simulink model "IF"  (R2024a)
settings: Solver=FixedStepAuto  StartTime=0.0  StopTime=5  FixedStep=1e-4  RelTol=1e-3
values from neighbouring files (symbols this model uses):
  Kt = 0.132    [IF.sldd]
  Pn = 8.0    [IF.sldd]
  Udc = 48.0    [IF.sldd]
undefined symbols (not defined in the file or in its folder): curr_d_ki, curr_d_kp, curr_q_ki, curr_q_kp, DiscIntNeverNeededParam
libraries: slpidlib x6, mcbplantlib x3, autolibpmsmexterior x3
(part 1 of 2)
settings Model: DataDictionary=IF.sldd  Creator=Administrator  LastModifiedBy=WuHongrui
settings OptimizationCC: DefaultParameterBehavior=Inlined  UseDivisionForNetSlopeComputation=on  GainParamInheritBuiltInType=on  UseFloatMulNetSlope=on  InlineInvariantSignals=on  PassReuseOutputArgsAs=Individual arguments  ZeroExternalMemoryAtStartup=off  ZeroInternalMemoryAtStartup=off  NoFixptDivByZeroProtection=on  EfficientFloat2IntCast=on  LifeSpan=1  OptimizeBlockOrder=speed  DifferentSizesBufferReuse=on  EfficientTunableParamExpr=on
settings DebuggingCC: ParameterTunabilityLossMsg=error  UnconnectedInputMsg=warning  UnconnectedOutputMsg=warning  UnconnectedLineMsg=warning
settings HardwareCC: ProdBitPerPointer=32  ProdBitPerSizeT=32  ProdBitPerPtrDiffT=32  ProdLargestAtomicInteger=Long  ProdLargestAtomicFloat=Double  ProdWordSize=32  ProdLongLongMode=on  ProdHWDeviceType=ARM Compatible->ARM Cortex-M
settings ModelReferenceCC: EnableRefExpFcnMdlSchedulingChecks=on
settings SFSimCC: MATLABDynamicMemAlloc=off
settings RTWCC: Description=Embedded Coder  SystemTargetFile=ert.tlc  GenCodeOnly=on  TemplateMakefile=ert_default_tmf  GenerateReport=on  LaunchReport=on  GenerateCodeReplacementReport=on  GPUComputeCapability=3.5  DLArmComputeVersion=19.05
settings CodeAppCC: ForceParamTrailComments=on  IgnoreCustomStorageClasses=off  OperatorAnnotations=on  SimulinkDataObjDesc=on  SFDataObjDesc=on  CustomSymbolStrGlobalVar=rt$N$M  CustomSymbolStrType=$N$M  CustomSymbolStrFcn=$N$M$F  CustomSymbolStrMacro=$N$M  InsertBlockDesc=on
settings ERTTargetCC: TargetLangStandard=C99 (ISO)  CodeReplacementLibrary=ARM Cortex-M  IncludeMdlTerminateFcn=off  CombineSignalStateStructs=on  SupportComplex=off  SupportNonInlinedSFcns=on  InlinedParameterPlacement=NonHierarchical  ERTCustomFileTemplate=example_file_process.tlc  ERTFilePackagingFormat=CompactWithDataFile

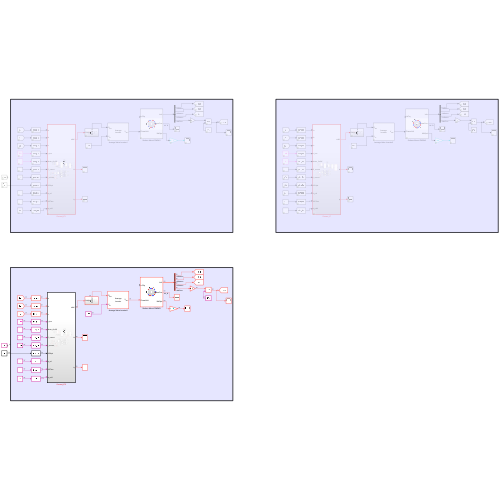
[thumbnail: Simulink's stored preview of the top-level diagram]
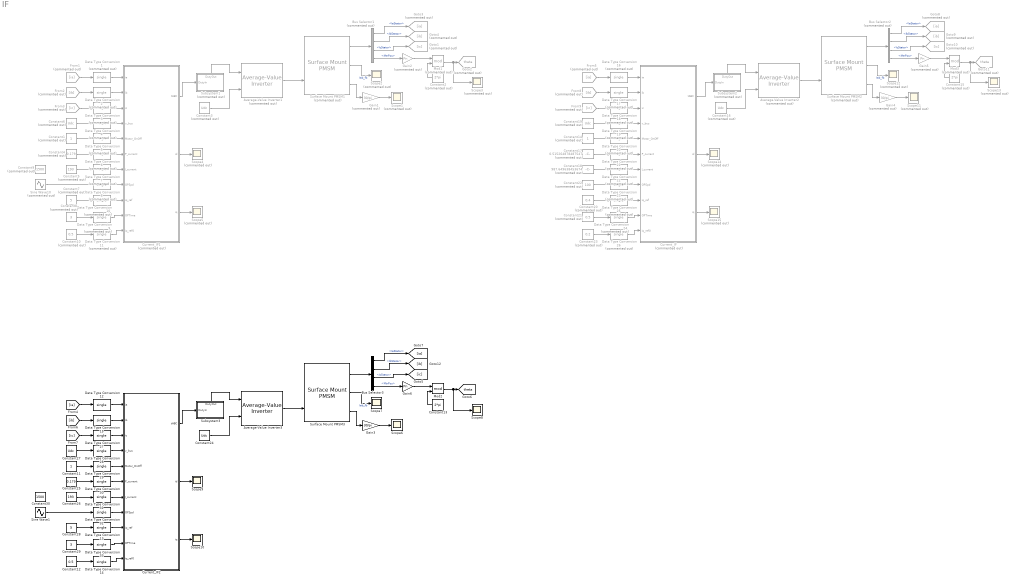
== system IF ==
  Average-Value Inverter1 : mcbplantlib/Average-Value Inverter  Commented=on
  Average-Value Inverter2 : mcbplantlib/Average-Value Inverter  Commented=on
  Average-Value Inverter3 : mcbplantlib/Average-Value Inverter
  Bus Selector1 : BusSelector  Commented=on  OutputSignals=IaStator,IbStator,IcStator,MtrPos
  Bus Selector2 : BusSelector  Commented=on  OutputSignals=IaStator,IbStator,IcStator,MtrPos
  Bus Selector3 : BusSelector  OutputSignals=IaStator,IbStator,IcStator,MtrPos
  Constant1 : Constant  Commented=on  OutDataTypeStr=single
  Constant10 : Constant  Commented=on  Value=0.5  OutDataTypeStr=single
  Constant11 : Constant  OutDataTypeStr=single
  Constant12 : Constant  Value=0.5  OutDataTypeStr=single
  Constant13 : Constant  Value=2*pi  OutDataTypeStr=single
  Constant14 : Constant  Commented=on  OutDataTypeStr=single
  Constant15 : Constant  Commented=on  Value=2*pi  OutDataTypeStr=single
  Constant16 : Constant  Commented=on  Value=Udc
  Constant17 : Constant  Commented=on  Value=0.515264878487547  OutDataTypeStr=single
  Constant18 : Constant  Commented=on  Value=987.649638453674  OutDataTypeStr=single
  Constant19 : Constant  Commented=on  Value=Udc  OutDataTypeStr=single
  Constant2 : Constant  Commented=on  Value=2*pi  OutDataTypeStr=single
  Constant20 : Constant  Commented=on  Value=0.4  OutDataTypeStr=single
  Constant21 : Constant  Commented=on  Value=0.5  OutDataTypeStr=single
  Constant22 : Constant  Commented=on  Value=100  OutDataTypeStr=single
  Constant23 : Constant  Commented=on  Value=0.2  OutDataTypeStr=single
  Constant24 : Constant  Value=Udc
  Constant25 : Constant  Value=0.179  OutDataTypeStr=single
  Constant26 : Constant  Value=193  OutDataTypeStr=single
  Constant27 : Constant  Value=Udc  OutDataTypeStr=single
  Constant28 : Constant  Value=5  OutDataTypeStr=single
  Constant29 : Constant  Value=3  OutDataTypeStr=single
  Constant3 : Constant  Commented=on  Value=Udc
  Constant30 : Constant  Value=1500  OutDataTypeStr=single
  Constant4 : Constant  Commented=on  Value=0.179  OutDataTypeStr=single
  Constant5 : Constant  Commented=on  Value=193  OutDataTypeStr=single
  Constant6 : Constant  Commented=on  Value=Udc  OutDataTypeStr=single
  Constant7 : Constant  Commented=on  Value=5  OutDataTypeStr=single
  Constant8 : Constant  Commented=on  Value=3  OutDataTypeStr=single
  Constant9 : Constant  Commented=on  Value=1500  OutDataTypeStr=single
  Current_IF : Subsystem  Commented=on  TreatAsAtomicUnit=on
  Current_IF1 : Subsystem  Commented=on  TreatAsAtomicUnit=on
  Current_IF2 : Subsystem  TreatAsAtomicUnit=on
  Data Type Conversion{1..11,16..26} (22 alike) : DataTypeConversion  Commented=on  OutDataTypeStr=single  SaturateOnIntegerOverflow=off  RndMeth=Floor
  Data Type Conversion{12..15,27..33} (11 alike) : DataTypeConversion  OutDataTypeStr=single  SaturateOnIntegerOverflow=off  RndMeth=Floor
  From1 : From  Commented=on  GotoTag=ia
  From2 : From  Commented=on  GotoTag=ib
  From3 : From  Commented=on  GotoTag=ic
  From5 : From  Commented=on  GotoTag=ia
  From8 : From  Commented=on  GotoTag=ib
  From9 : From  Commented=on  GotoTag=ic
  Gain1 : Gain  Commented=on  Gain=30/pi  OutDataTypeStr=single
  Gain2 : Gain  Commented=on  Gain=Pn  OutDataTypeStr=single
  Gain3 : Gain  Gain=30/pi  OutDataTypeStr=single
  Gain4 : Gain  Commented=on  Gain=30/pi  OutDataTypeStr=single
  Gain5 : Gain  Commented=on  Gain=Pn  OutDataTypeStr=single
  Gain6 : Gain  Gain=Pn  OutDataTypeStr=single
  Goto1 : Goto  Commented=on  GotoTag=ic
  Goto10 : Goto  Commented=on  GotoTag=ic
  Goto11 : Goto  Commented=on  GotoTag=theta  TagVisibility=global
  Goto2 : Goto  Commented=on  GotoTag=theta  TagVisibility=global
  Goto3 : Goto  Commented=on  GotoTag=ia
  Goto4 : Goto  Commented=on  GotoTag=ib
  Goto8 : Goto  Commented=on  GotoTag=ia
  Goto9 : Goto  Commented=on  GotoTag=ib
  Mod1 : Math  Commented=on  Operator=mod  OutputSignalType=real
  Mod2 : Math  Operator=mod  OutputSignalType=real
  Mod3 : Math  Commented=on  Operator=mod  OutputSignalType=real
  Scope{1..5,11..15} (10 alike) : Scope  Commented=on
  Scope{6..10} (5 alike) : Scope
  Sine Wave1 : Sin  Amplitude=500  Frequency=5  SampleTime=0
  Sine Wave10 : Sin  Commented=on  Amplitude=500  Frequency=5  SampleTime=0
  Subsystem1 : Subsystem  Commented=on
      settings: PortSchema="{\"entries\":[{\"content\":{\"sides\":[{\"content\":{\"connectorIds\":[\"In1\"]},\"type\":\"ConnectorPlacement.EquallySpacedRectSide\",\"uuid\":\"8ccc51de-fa2a-4900-80a3-4cdf9aa76f01\"},{\"content\":{\"connectorIds\":[],\"side\":\"RIGHT\"},\"type\":\"ConnectorPlacement.EquallySpacedRectSide\",\"uuid\":\"32c06e0d-3f1d-4948-af96-e310e54308a0\"},{\"content\":{\"connectorIds\":[\"Out1\"],\"side\":\"TOP\"},\"type\":\"ConnectorPlacement.EquallySpacedRectSide\",\"uuid\":\"a9066067-2c54-42a8-b4d7-fb86ac71b860\"}]},\"type\":\"ConnectorPlacement.EquallySpacedConnector\",\"uuid\":\"e4576975-acad-4e16-822f-2c2e7f23d7a7\"}],\"packageUris\":[\"http://schema.mathworks.com/mf0/Connector/R2020b\"],\"version\":\"1.0\"}"
  Subsystem2 : Subsystem  Commented=on
      settings: PortSchema="{\"entries\":[{\"content\":{\"sides\":[{\"content\":{\"connectorIds\":[\"In1\"]},\"type\":\"ConnectorPlacement.EquallySpacedRectSide\",\"uuid\":\"8ccc51de-fa2a-4900-80a3-4cdf9aa76f01\"},{\"content\":{\"connectorIds\":[],\"side\":\"RIGHT\"},\"type\":\"ConnectorPlacement.EquallySpacedRectSide\",\"uuid\":\"32c06e0d-3f1d-4948-af96-e310e54308a0\"},{\"content\":{\"connectorIds\":[\"Out1\"],\"side\":\"TOP\"},\"type\":\"ConnectorPlacement.EquallySpacedRectSide\",\"uuid\":\"a9066067-2c54-42a8-b4d7-fb86ac71b860\"}]},\"type\":\"ConnectorPlacement.EquallySpacedConnector\",\"uuid\":\"e4576975-acad-4e16-822f-2c2e7f23d7a7\"}],\"packageUris\":[\"http://schema.mathworks.com/mf0/Connector/R2020b\"],\"version\":\"1.0\"}"
  Subsystem3 : Subsystem
      settings: PortSchema="{\"entries\":[{\"content\":{\"sides\":[{\"content\":{\"connectorIds\":[\"In1\"]},\"type\":\"ConnectorPlacement.EquallySpacedRectSide\",\"uuid\":\"8ccc51de-fa2a-4900-80a3-4cdf9aa76f01\"},{\"content\":{\"connectorIds\":[],\"side\":\"RIGHT\"},\"type\":\"ConnectorPlacement.EquallySpacedRectSide\",\"uuid\":\"32c06e0d-3f1d-4948-af96-e310e54308a0\"},{\"content\":{\"connectorIds\":[\"Out1\"],\"side\":\"TOP\"},\"type\":\"ConnectorPlacement.EquallySpacedRectSide\",\"uuid\":\"a9066067-2c54-42a8-b4d7-fb86ac71b860\"}]},\"type\":\"ConnectorPlacement.EquallySpacedConnector\",\"uuid\":\"e4576975-acad-4e16-822f-2c2e7f23d7a7\"}],\"packageUris\":[\"http://schema.mathworks.com/mf0/Connector/R2020b\"],\"version\":\"1.0\"}"
  Surface Mount PMSM1 : autolibpmsmexterior/Surface Mount PMSM  Commented=on  port_config=Torque  sim_type=Discrete  Ts=1e-4  P=Pn  Rs=Rs  Ldq_=L  KConstText=Torque constant (Kt):  lambda_pm=flux  Ke=0.0059268  Kt=Kt  mechanical=[0.096e-4, 2e-5, 0]  idq0=[0 0]  theta_init=0  omega_init=0  KConst=Kt  lambda_pm_calc=0.011  RefBlkName='autolibpmsmexterior/Surface Mount PMSM'  aMode=5  Ldq="[0.0017      0.0017]"
  Surface Mount PMSM2 : autolibpmsmexterior/Surface Mount PMSM  Commented=on  port_config=Torque  sim_type=Discrete  Ts=1e-4  P=Pn  Rs=Rs  Ldq_=L  KConstText=Torque constant (Kt):  lambda_pm=flux  Ke=0.0059268  Kt=Kt  mechanical=[0.096e-4, 2e-5, 0]  idq0=[0 0]  theta_init=0  omega_init=0  KConst=Kt  lambda_pm_calc=0.011  RefBlkName='autolibpmsmexterior/Surface Mount PMSM'  aMode=5  Ldq="[0.0017      0.0017]"
  Surface Mount PMSM3 : autolibpmsmexterior/Surface Mount PMSM  port_config=Torque  sim_type=Discrete  Ts=1e-4  P=Pn  Rs=Rs  Ldq_=L  KConstText=Torque constant (Kt):  lambda_pm=flux  Ke=0.0059268  Kt=Kt  mechanical=[0.096e-4, 2e-5, 0]  idq0=[0 0]  theta_init=0  omega_init=0  KConst=Kt  lambda_pm_calc=0.011  RefBlkName='autolibpmsmexterior/Surface Mount PMSM'  aMode=5  Ldq="[0.0017      0.0017]"
  tag scope: theta=global
  wires:
  Data Type Conversion18/1 -> Current_IF/3(ic)
  Current_IF/3(iq) -> Scope15/1
  Gain4/1 -> Scope11/1
  Constant16/1 -> Average-Value Inverter2/2
  From8/1 -> Data Type Conversion17/1
  Data Type Conversion16/1 -> Current_IF/1(ia)
  Bus Selector2/4 -> Gain5/1  "<MtrPos>"
  Constant17/1 -> Data Type Conversion21/1
  Constant18/1 -> Data Type Conversion22/1
  Data Type Conversion19/1 -> Current_IF/4(v_bus)
  Constant19/1 -> Data Type Conversion19/1
  Data Type Conversion21/1 -> Current_IF/6(P_current)
  Current_IF/2(id) -> Scope14/1
  Current_IF/1(tABC) -> Subsystem2/1(DutyIn)
  Data Type Conversion20/1 -> Current_IF/5(Motor_OnOff)
  Data Type Conversion22/1 -> Current_IF/7(I_current)
  Bus Selector2/1 -> Goto8/1  "<IaStator>"
  Average-Value Inverter2/1 -> Surface Mount PMSM2/2
  From9/1 -> Data Type Conversion18/1
  Bus Selector2/2 -> Goto9/1  "<IbStator>"
  Constant14/1 -> Data Type Conversion20/1
  Subsystem2/1(DutyOut) -> Average-Value Inverter2/1
  Constant15/1 -> Mod3/2
  Mod3/1 -> Scope13/1, Goto11/1
  From5/1 -> Data Type Conversion16/1
  Surface Mount PMSM2/3 -> Gain4/1
  Gain5/1 -> Mod3/1
  Bus Selector2/3 -> Goto10/1  "<IcStator>"
  Surface Mount PMSM2/1 -> Bus Selector2/1
  Data Type Conversion17/1 -> Current_IF/2(ib)
  Surface Mount PMSM2/2 -> Scope12/1  "Iab_fb"
  Data Type Conversion23/1 -> Current_IF/8(OPSpd)
  Constant22/1 -> Data Type Conversion23/1
  Data Type Conversion25/1 -> Current_IF/9(iq_ref)
  Constant20/1 -> Data Type Conversion25/1
  Constant21/1 -> Data Type Conversion24/1
  Data Type Conversion24/1 -> Current_IF/10(OPTime)
  Constant23/1 -> Data Type Conversion26/1
  Data Type Conversion26/1 -> Current_IF/11(iq_ref0)
  Current_IF1/1(tABC) -> Subsystem1/1(DutyIn)
  Bus Selector1/2 -> Goto4/1  "<IbStator>"
  Gain1/1 -> Scope1/1
  Data Type Conversion3/1 -> Current_IF1/3(ic)
  From2/1 -> Data Type Conversion2/1
  Constant3/1 -> Average-Value Inverter1/2
  Constant1/1 -> Data Type Conversion5/1
  Constant5/1 -> Data Type Conversion7/1
  Current_IF1/2(id) -> Scope4/1
  Constant4/1 -> Data Type Conversion6/1
  Data Type Conversion6/1 -> Current_IF1/6(P_current)
  Bus Selector1/4 -> Gain2/1  "<MtrPos>"
  Data Type Conversion1/1 -> Current_IF1/1(ia)
  Current_IF1/3(iq) -> Scope5/1
  From3/1 -> Data Type Conversion3/1
  Surface Mount PMSM1/3 -> Gain1/1
  Constant10/1 -> Data Type Conversion11/1
  Bus Selector1/1 -> Goto3/1  "<IaStator>"
  Average-Value Inverter1/1 -> Surface Mount PMSM1/2
  Constant2/1 -> Mod1/2
  Constant7/1 -> Data Type Conversion10/1
  Data Type Conversion5/1 -> Current_IF1/5(Motor_OnOff)
  Constant8/1 -> Data Type Conversion9/1
  Data Type Conversion8/1 -> Current_IF1/8(OPSpd)
  Gain2/1 -> Mod1/1
  Data Type Conversion2/1 -> Current_IF1/2(ib)
  Surface Mount PMSM1/2 -> Scope2/1  "Iab_fb"
  Subsystem1/1(DutyOut) -> Average-Value Inverter1/1
  Data Type Conversion10/1 -> Current_IF1/9(iq_ref)
  Data Type Conversion7/1 -> Current_IF1/7(I_current)
  Data Type Conversion4/1 -> Current_IF1/4(v_bus)
  Constant6/1 -> Data Type Conversion4/1
  Sine Wave10/1 -> Data Type Conversion8/1
  Bus Selector1/3 -> Goto1/1  "<IcStator>"
  Data Type Conversion9/1 -> Current_IF1/10(OPTime)
  Surface Mount PMSM1/1 -> Bus Selector1/1
  Mod1/1 -> Scope3/1, Goto2/1
  Data Type Conversion11/1 -> Current_IF1/11(iq_ref0)
  From1/1 -> Data Type Conversion1/1
  Constant11/1 -> Data Type Conversion29/1
  Constant26/1 -> Data Type Conversion31/1
  Constant25/1 -> Data Type Conversion30/1
  Data Type Conversion27/1 -> Current_IF2/3(ic)
  Surface Mount PMSM3/1 -> Bus Selector3/1
  [ib] -> Data Type Conversion15/1
  Data Type Conversion14/1 -> Current_IF2/11(iq_ref0)
  Data Type Conversion12/1 -> Current_IF2/1(ia)
  Mod2/1 -> Scope8/1, [theta]
  Subsystem3/1(DutyOut) -> Average-Value Inverter3/1
  Constant28/1 -> Data Type Conversion13/1
  Data Type Conversion33/1 -> Current_IF2/10(OPTime)
  Constant13/1 -> Mod2/2
  [ia] -> Data Type Conversion12/1
  Bus Selector3/3 -> [ic]  "<IcStator>"
  Current_IF2/2(id) -> Scope9/1
  Current_IF2/3(iq) -> Scope10/1
  Sine Wave1/1 -> Data Type Conversion32/1
  Current_IF2/1(tABC) -> Subsystem3/1(DutyIn)
  Constant27/1 -> Data Type Conversion28/1
  Data Type Conversion15/1 -> Current_IF2/2(ib)
  Surface Mount PMSM3/2 -> Scope7/1  "Iab_fb"
  Data Type Conversion30/1 -> Current_IF2/6(P_current)
  Constant24/1 -> Average-Value Inverter3/2
  Bus Selector3/4 -> Gain6/1  "<MtrPos>"
  Bus Selector3/2 -> [ib]  "<IbStator>"
  [ic] -> Data Type Conversion27/1
  Gain6/1 -> Mod2/1
  Data Type Conversion28/1 -> Current_IF2/4(v_bus)
  Constant29/1 -> Data Type Conversion33/1
  Constant12/1 -> Data Type Conversion14/1
  Data Type Conversion29/1 -> Current_IF2/5(Motor_OnOff)
  Surface Mount PMSM3/3 -> Gain3/1
  Bus Selector3/1 -> [ia]  "<IaStator>"
  Average-Value Inverter3/1 -> Surface Mount PMSM3/2
  Gain3/1 -> Scope6/1
  Data Type Conversion32/1 -> Current_IF2/8(OPSpd)
  Data Type Conversion31/1 -> Current_IF2/7(I_current)
  Data Type Conversion13/1 -> Current_IF2/9(iq_ref)

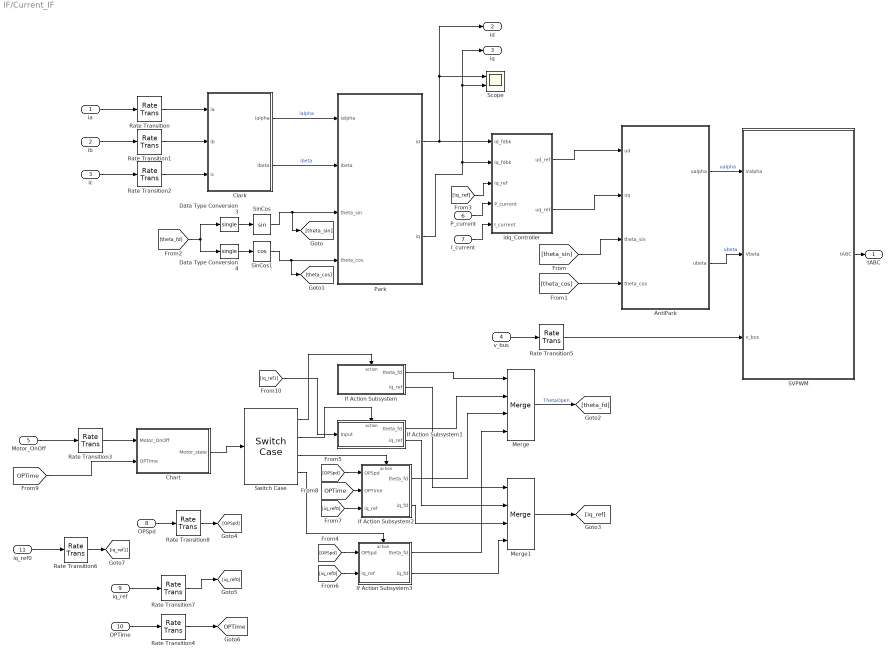
== system IF/Current_IF ==
  ia : Inport
  ib : Inport  Port=2
  ic : Inport  Port=3
  v_bus : Inport  Port=4
  Motor_OnOff : Inport  Port=5
  P_current : Inport  Port=6
  I_current : Inport  Port=7
  OPSpd : Inport  Port=8
  iq_ref : Inport  Port=9
  OPTime : Inport  Port=10
  iq_ref0 : Inport  Port=11
  AntiPark : Subsystem
  Chart : Stateflow chart  TreatAsAtomicUnit=on
  Clark : Subsystem
  Data Type Conversion3 : DataTypeConversion  OutDataTypeStr=single  SaturateOnIntegerOverflow=off  RndMeth=Floor
  Data Type Conversion4 : DataTypeConversion  OutDataTypeStr=single  SaturateOnIntegerOverflow=off  RndMeth=Floor
  If Action Subsystem : Subsystem  TreatAsAtomicUnit=on
  If Action Subsystem1 : Subsystem  TreatAsAtomicUnit=on
  If Action Subsystem2 : Subsystem  TreatAsAtomicUnit=on
  If Action Subsystem3 : Subsystem  TreatAsAtomicUnit=on
  Merge : Merge  Inputs=4
  Merge1 : Merge  Inputs=4
  Park : Subsystem
  Rate Transition{,1..8} (9 alike) : RateTransition
  SVPWM : Subsystem  TreatAsAtomicUnit=on
  Scope : Scope  NumInputPorts=2
  SinCos : Trigonometry
  SinCos1 : Trigonometry  Operator=cos
  Switch Case : SwitchCase  CaseConditions={1,2,3,4}  ShowDefaultCase=off
  idq_Controller : Subsystem
  tABC : Outport
  id : Outport  Port=2
  iq : Outport  Port=3
  tag scope: OPTime=global
  wires:
  Data Type Conversion4/1 -> SinCos1/1
  Data Type Conversion3/1 -> SinCos/1
  AntiPark/2(ubeta) -> SVPWM/2(Vbeta)  "ubeta"
  AntiPark/1(ualpha) -> SVPWM/1(Valpha)  "ualpha"
  [theta_cos] -> AntiPark/4(theta_cos)
  [theta_sin] -> AntiPark/3(theta_sin)
  SinCos/1 -> Park/3(theta_sin), [theta_sin]
  [theta_fd] -> Data Type Conversion3/1, Data Type Conversion4/1
  SinCos1/1 -> Park/4(theta_cos), [theta_cos]
  v_bus/1 -> Rate Transition5/1
  SVPWM/1(tABC) -> tABC/1
  ib/1 -> Rate Transition1/1
  ia/1 -> Rate Transition/1
  ic/1 -> Rate Transition2/1
  Clark/1(ialpha) -> Park/1(ialpha)  "ialpha"
  Clark/2(ibeta) -> Park/2(ibeta)  "ibeta"
  idq_Controller/1(ud_ref) -> AntiPark/1(ud)
  idq_Controller/2(uq_ref) -> AntiPark/2(uq)
  Park/1(id) -> id/1, Scope/1, idq_Controller/1(id_fdbk)
  Park/2(iq) -> Scope/2, iq/1, idq_Controller/2(iq_fdbk)
  [iq_ref] -> idq_Controller/3(iq_ref)
  [OPSpd] -> If Action Subsystem2/1(OPSpd)
  [iq_ref0] -> If Action Subsystem3/2(iq_ref)
  Switch Case/2 -> If Action Subsystem1/Action
  Chart/1(Motor_state) -> Switch Case/1
  [OPSpd] -> If Action Subsystem3/1(OPSpd)
  Switch Case/4 -> If Action Subsystem3/Action
  [OPTime] -> If Action Subsystem2/2(OPTime)
  [iq_ref0] -> If Action Subsystem2/3(iq_ref)
  Switch Case/1 -> If Action Subsystem/Action
  Switch Case/3 -> If Action Subsystem2/Action
  If Action Subsystem/1(theta_fd) -> Merge/1
  If Action Subsystem1/1(theta_fd) -> Merge/2
  If Action Subsystem2/1(theta_fd) -> Merge/3
  If Action Subsystem3/1(theta_fd) -> Merge/4
  If Action Subsystem/2(iq_ref) -> Merge1/1
  If Action Subsystem1/2(iq_ref) -> Merge1/2
  If Action Subsystem2/2(iq_fd) -> Merge1/3
  If Action Subsystem3/2(iq_fd) -> Merge1/4
  Merge/1 -> [theta_fd]  "ThetaOpen"
  Merge1/1 -> [iq_ref]
  Motor_OnOff/1 -> Rate Transition3/1
  P_current/1 -> idq_Controller/4(P_current)
  I_current/1 -> idq_Controller/5(I_current)
  Rate Transition/1 -> Clark/1(ia)
  Rate Transition1/1 -> Clark/2(ib)
  Rate Transition2/1 -> Clark/3(ic)
  Rate Transition5/1 -> SVPWM/3(v_bus)
  OPTime/1 -> Rate Transition4/1
  Rate Transition3/1 -> Chart/1(Motor_OnOff)
  Rate Transition4/1 -> [OPTime]
  [OPTime] -> Chart/2(OPTime)
  iq_ref0/1 -> Rate Transition6/1
  [iq_ref1] -> If Action Subsystem1/1(Input)
  Rate Transition6/1 -> [iq_ref1]
  iq_ref/1 -> Rate Transition7/1
  Rate Transition7/1 -> [iq_ref0]
  Rate Transition8/1 -> [OPSpd]
  OPSpd/1 -> Rate Transition8/1

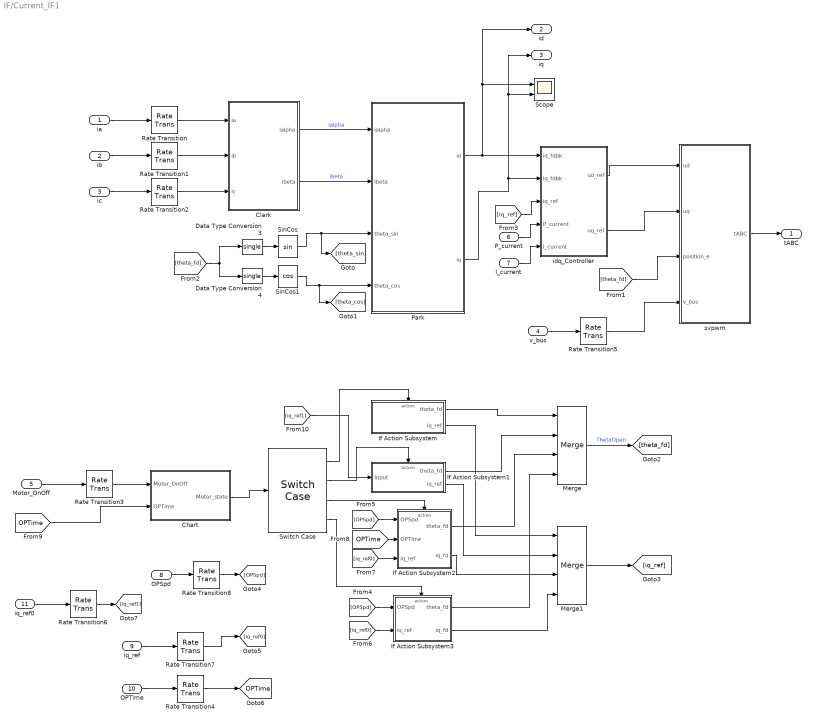
== system IF/Current_IF1 ==
  ia : Inport
  ib : Inport  Port=2
  ic : Inport  Port=3
  v_bus : Inport  Port=4
  Motor_OnOff : Inport  Port=5
  P_current : Inport  Port=6
  I_current : Inport  Port=7
  OPSpd : Inport  Port=8
  iq_ref : Inport  Port=9
  OPTime : Inport  Port=10
  iq_ref0 : Inport  Port=11
  Chart : Stateflow chart  TreatAsAtomicUnit=on
  Clark : Subsystem
  Data Type Conversion3 : DataTypeConversion  OutDataTypeStr=single  SaturateOnIntegerOverflow=off  RndMeth=Floor
  Data Type Conversion4 : DataTypeConversion  OutDataTypeStr=single  SaturateOnIntegerOverflow=off  RndMeth=Floor
  If Action Subsystem : Subsystem  TreatAsAtomicUnit=on
  If Action Subsystem1 : Subsystem  TreatAsAtomicUnit=on
  If Action Subsystem2 : Subsystem  TreatAsAtomicUnit=on
  If Action Subsystem3 : Subsystem  TreatAsAtomicUnit=on
  Merge : Merge  Inputs=4
  Merge1 : Merge  Inputs=4
  Park : Subsystem
  Rate Transition{,1..8} (9 alike) : RateTransition
  Scope : Scope  NumInputPorts=2
  SinCos : Trigonometry
  SinCos1 : Trigonometry  Operator=cos
  Switch Case : SwitchCase  CaseConditions={1,2,3,4}  ShowDefaultCase=off
  idq_Controller : Subsystem
  svpwm : Subsystem
  tABC : Outport
  id : Outport  Port=2
  iq : Outport  Port=3
  tag scope: OPTime=global
  wires:
  Data Type Conversion4/1 -> SinCos1/1
  Data Type Conversion3/1 -> SinCos/1
  SinCos/1 -> Park/3(theta_sin), [theta_sin]
  [theta_fd] -> Data Type Conversion3/1, Data Type Conversion4/1
  SinCos1/1 -> Park/4(theta_cos), [theta_cos]
  v_bus/1 -> Rate Transition5/1
  ib/1 -> Rate Transition1/1
  ia/1 -> Rate Transition/1
  ic/1 -> Rate Transition2/1
  Clark/1(ialpha) -> Park/1(ialpha)  "ialpha"
  Clark/2(ibeta) -> Park/2(ibeta)  "ibeta"
  Park/1(id) -> id/1, Scope/1, idq_Controller/1(id_fdbk)
  Park/2(iq) -> Scope/2, iq/1, idq_Controller/2(iq_fdbk)
  [iq_ref] -> idq_Controller/3(iq_ref)
  [OPSpd] -> If Action Subsystem2/1(OPSpd)
  [iq_ref0] -> If Action Subsystem3/2(iq_ref)
  Switch Case/2 -> If Action Subsystem1/Action
  Chart/1(Motor_state) -> Switch Case/1
  [OPSpd] -> If Action Subsystem3/1(OPSpd)
  Switch Case/4 -> If Action Subsystem3/Action
  [OPTime] -> If Action Subsystem2/2(OPTime)
  [iq_ref0] -> If Action Subsystem2/3(iq_ref)
  Switch Case/1 -> If Action Subsystem/Action
  Switch Case/3 -> If Action Subsystem2/Action
  If Action Subsystem/1(theta_fd) -> Merge/1
  If Action Subsystem1/1(theta_fd) -> Merge/2
  If Action Subsystem2/1(theta_fd) -> Merge/3
  If Action Subsystem3/1(theta_fd) -> Merge/4
  If Action Subsystem/2(iq_ref) -> Merge1/1
  If Action Subsystem1/2(iq_ref) -> Merge1/2
  If Action Subsystem2/2(iq_fd) -> Merge1/3
  If Action Subsystem3/2(iq_fd) -> Merge1/4
  Merge/1 -> [theta_fd]  "ThetaOpen"
  Merge1/1 -> [iq_ref]
  Motor_OnOff/1 -> Rate Transition3/1
  P_current/1 -> idq_Controller/4(P_current)
  I_current/1 -> idq_Controller/5(I_current)
  Rate Transition/1 -> Clark/1(ia)
  Rate Transition1/1 -> Clark/2(ib)
  Rate Transition2/1 -> Clark/3(ic)
  OPTime/1 -> Rate Transition4/1
  Rate Transition3/1 -> Chart/1(Motor_OnOff)
  Rate Transition4/1 -> [OPTime]
  [OPTime] -> Chart/2(OPTime)
  iq_ref0/1 -> Rate Transition6/1
  [iq_ref1] -> If Action Subsystem1/1(Input)
  Rate Transition6/1 -> [iq_ref1]
  iq_ref/1 -> Rate Transition7/1
  Rate Transition7/1 -> [iq_ref0]
  Rate Transition8/1 -> [OPSpd]
  OPSpd/1 -> Rate Transition8/1
  idq_Controller/1(ud_ref) -> svpwm/1(ud)
  idq_Controller/2(uq_ref) -> svpwm/2(uq)
  Rate Transition5/1 -> svpwm/4(v_bus)
  svpwm/1(tABC) -> tABC/1
  [theta_fd] -> svpwm/3(position_e)

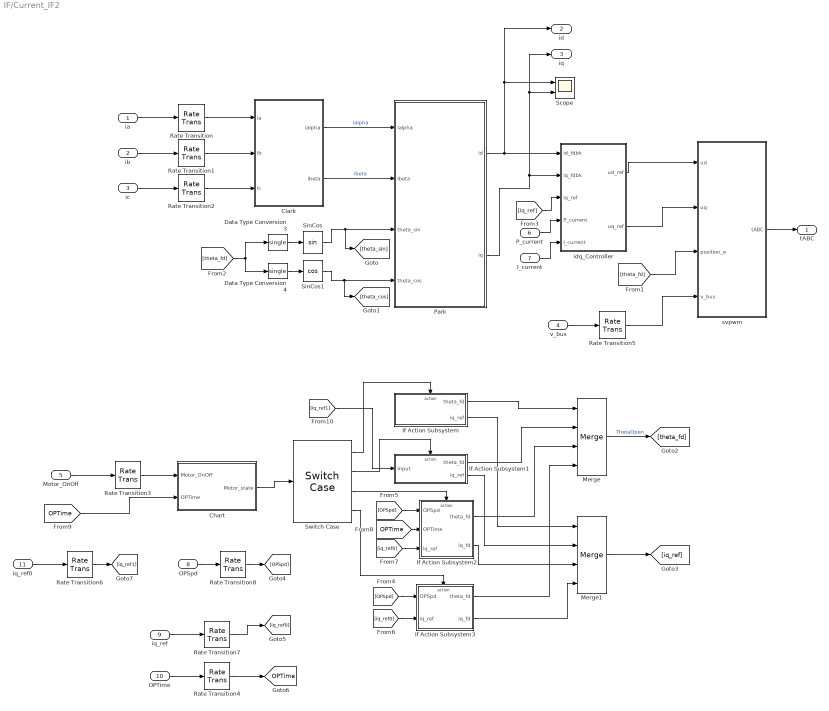
== system IF/Current_IF2 ==
  ia : Inport
  ib : Inport  Port=2
  ic : Inport  Port=3
  v_bus : Inport  Port=4
  Motor_OnOff : Inport  Port=5
  P_current : Inport  Port=6
  I_current : Inport  Port=7
  OPSpd : Inport  Port=8
  iq_ref : Inport  Port=9
  OPTime : Inport  Port=10
  iq_ref0 : Inport  Port=11
  Chart : Stateflow chart  TreatAsAtomicUnit=on
  Clark : Subsystem
  Data Type Conversion3 : DataTypeConversion  OutDataTypeStr=single  SaturateOnIntegerOverflow=off  RndMeth=Floor
  Data Type Conversion4 : DataTypeConversion  OutDataTypeStr=single  SaturateOnIntegerOverflow=off  RndMeth=Floor
  If Action Subsystem : Subsystem  TreatAsAtomicUnit=on
  If Action Subsystem1 : Subsystem  TreatAsAtomicUnit=on
  If Action Subsystem2 : Subsystem  TreatAsAtomicUnit=on
  If Action Subsystem3 : Subsystem  TreatAsAtomicUnit=on
  Merge : Merge  Inputs=4
  Merge1 : Merge  Inputs=4
  Park : Subsystem
  Rate Transition{,1..8} (9 alike) : RateTransition
  Scope : Scope  NumInputPorts=2
  SinCos : Trigonometry
  SinCos1 : Trigonometry  Operator=cos
  Switch Case : SwitchCase  CaseConditions={1,2,3,4}  ShowDefaultCase=off
  idq_Controller : Subsystem
  svpwm : Subsystem
  tABC : Outport
  id : Outport  Port=2
  iq : Outport  Port=3
  tag scope: OPTime=global
  wires:
  Data Type Conversion4/1 -> SinCos1/1
  Data Type Conversion3/1 -> SinCos/1
  SinCos/1 -> Park/3(theta_sin), [theta_sin]
  [theta_fd] -> Data Type Conversion3/1, Data Type Conversion4/1
  SinCos1/1 -> Park/4(theta_cos), [theta_cos]
  v_bus/1 -> Rate Transition5/1
  ib/1 -> Rate Transition1/1
  ia/1 -> Rate Transition/1
  ic/1 -> Rate Transition2/1
  Clark/1(ialpha) -> Park/1(ialpha)  "ialpha"
  Clark/2(ibeta) -> Park/2(ibeta)  "ibeta"
  Park/1(id) -> id/1, Scope/1, idq_Controller/1(id_fdbk)
  Park/2(iq) -> Scope/2, iq/1, idq_Controller/2(iq_fdbk)
  [iq_ref] -> idq_Controller/3(iq_ref)
  [OPSpd] -> If Action Subsystem2/1(OPSpd)
  [iq_ref0] -> If Action Subsystem3/2(iq_ref)
  Switch Case/2 -> If Action Subsystem1/Action
  Chart/1(Motor_state) -> Switch Case/1
  [OPSpd] -> If Action Subsystem3/1(OPSpd)
  Switch Case/4 -> If Action Subsystem3/Action
  [OPTime] -> If Action Subsystem2/2(OPTime)
  [iq_ref0] -> If Action Subsystem2/3(iq_ref)
  Switch Case/1 -> If Action Subsystem/Action
  Switch Case/3 -> If Action Subsystem2/Action
  If Action Subsystem/1(theta_fd) -> Merge/1
  If Action Subsystem1/1(theta_fd) -> Merge/2
  If Action Subsystem2/1(theta_fd) -> Merge/3
  If Action Subsystem3/1(theta_fd) -> Merge/4
  If Action Subsystem/2(iq_ref) -> Merge1/1
  If Action Subsystem1/2(iq_ref) -> Merge1/2
  If Action Subsystem2/2(iq_fd) -> Merge1/3
  If Action Subsystem3/2(iq_fd) -> Merge1/4
  Merge/1 -> [theta_fd]  "ThetaOpen"
  Merge1/1 -> [iq_ref]
  Motor_OnOff/1 -> Rate Transition3/1
  P_current/1 -> idq_Controller/4(P_current)
  I_current/1 -> idq_Controller/5(I_current)
  Rate Transition/1 -> Clark/1(ia)
  Rate Transition1/1 -> Clark/2(ib)
  Rate Transition2/1 -> Clark/3(ic)
  OPTime/1 -> Rate Transition4/1
  Rate Transition3/1 -> Chart/1(Motor_OnOff)
  Rate Transition4/1 -> [OPTime]
  [OPTime] -> Chart/2(OPTime)
  iq_ref0/1 -> Rate Transition6/1
  [iq_ref1] -> If Action Subsystem1/1(Input)
  Rate Transition6/1 -> [iq_ref1]
  iq_ref/1 -> Rate Transition7/1
  Rate Transition7/1 -> [iq_ref0]
  Rate Transition8/1 -> [OPSpd]
  OPSpd/1 -> Rate Transition8/1
  idq_Controller/1(ud_ref) -> svpwm/1(ud)
  idq_Controller/2(uq_ref) -> svpwm/2(uq)
  Rate Transition5/1 -> svpwm/4(v_bus)
  svpwm/1(tABC) -> tABC/1
  [theta_fd] -> svpwm/3(position_e)

== system IF/Subsystem1 ==
  DutyIn : Inport
  Constant : Constant  Value=0.5  SampleTime=-1
  Gain : Gain  Gain=1/8000  ParamDataTypeStr=single
  Gain1 : Gain  Gain=-1
  Sum : Sum  Inputs=|+-
  Sum1 : Sum  Inputs=|++
  DutyOut : Outport
  wires:
  Sum/1 -> Gain1/1
  Constant/1 -> Sum1/2, Sum/2
  DutyIn/1 -> Gain/1
  Gain1/1 -> Sum1/1
  Sum1/1 -> DutyOut/1
  Gain/1 -> Sum/1

== system IF/Subsystem2 ==
  DutyIn : Inport
  Constant : Constant  Value=0.5  SampleTime=-1
  Gain : Gain  Gain=1/8000  ParamDataTypeStr=single
  Gain1 : Gain  Gain=-1
  Sum : Sum  Inputs=|+-
  Sum1 : Sum  Inputs=|++
  DutyOut : Outport
  wires:
  Sum/1 -> Gain1/1
  Constant/1 -> Sum1/2, Sum/2
  DutyIn/1 -> Gain/1
  Gain1/1 -> Sum1/1
  Sum1/1 -> DutyOut/1
  Gain/1 -> Sum/1

== system IF/Subsystem3 ==
  DutyIn : Inport
  Constant : Constant  Value=0.5  SampleTime=-1
  Gain : Gain  Gain=1/8000  ParamDataTypeStr=single
  Gain1 : Gain  Gain=-1
  Sum : Sum  Inputs=|+-
  Sum1 : Sum  Inputs=|++
  DutyOut : Outport
  wires:
  Sum/1 -> Gain1/1
  Constant/1 -> Sum1/2, Sum/2
  DutyIn/1 -> Gain/1
  Gain1/1 -> Sum1/1
  Sum1/1 -> DutyOut/1
  Gain/1 -> Sum/1

== system IF/Current_IF/AntiPark ==
  note: Valpha = ud*cos(theta) - uq*sin(theta);
      | Vbeta = ud*sin(theta) + uq*cos(theta);
  ud : Inport
  uq : Inport  Port=2
  theta_sin : Inport  Port=3
  theta_cos : Inport  Port=4
  Add : Sum  Inputs=+-
  Add1 : Sum
  Product{,1..3} (4 alike) : Product
  ualpha : Outport  OutDataTypeStr=single
  ubeta : Outport  Port=2  OutDataTypeStr=single
  wires:
  Product2/1 -> Add1/1
  Product/1 -> Add/1
  Add/1 -> ualpha/1
  Product3/1 -> Add1/2
  ud/1 -> Product/1, Product2/1
  theta_sin/1 -> Product1/2, Product2/2
  theta_cos/1 -> Product3/2, Product/2
  uq/1 -> Product1/1, Product3/1
  Product1/1 -> Add/2
  Add1/1 -> ubeta/1

== system IF/Current_IF/Clark ==
  note: ialpha = ia*2/3-(ib+ic)/3;
      | ibeta = (ib-ic)*sqrt(3)/3;
  ia : Inport  OutDataTypeStr=single
  ib : Inport  Port=2  OutDataTypeStr=single
  ic : Inport  Port=3  OutDataTypeStr=single
  Add : Sum  OutDataTypeStr=single  AccumDataTypeStr=single
  Add1 : Sum  Inputs=+-  OutDataTypeStr=single  AccumDataTypeStr=single
  Add2 : Sum  Inputs=+-  OutDataTypeStr=single  AccumDataTypeStr=single
  Gain : Gain  Gain=2/3  ParamDataTypeStr=single
  Gain1 : Gain  Gain=1/3  ParamDataTypeStr=single
  Gain2 : Gain  Gain=sqrt(3)/3  ParamDataTypeStr=single
  ialpha : Outport  OutDataTypeStr=single
  ibeta : Outport  Port=2  OutDataTypeStr=single
  wires:
  Add1/1 -> ialpha/1
  ia/1 -> Gain/1
  Gain2/1 -> ibeta/1
  ib/1 -> Add/1, Add2/1
  Gain/1 -> Add1/1
  Add2/1 -> Gain2/1
  Add/1 -> Gain1/1
  ic/1 -> Add/2, Add2/2
  Gain1/1 -> Add1/2

== system IF/Current_IF/If Action Subsystem ==
  Action Port : ActionPort  ActionPortLabel=case [ 1 ]:
  Constant : Constant  Value=0  OutDataTypeStr=single
  Constant1 : Constant  Value=0  OutDataTypeStr=single
  theta_fd : Outport
  iq_ref : Outport  Port=2
  wires:
  Constant1/1 -> iq_ref/1
  Constant/1 -> theta_fd/1

== system IF/Current_IF/If Action Subsystem1 ==
  Input : Inport
  Action Port : ActionPort  ActionPortLabel=case [ 2 ]:
  Constant : Constant  Value=0  OutDataTypeStr=single
  theta_fd : Outport
  iq_ref : Outport  Port=2
  wires:
  Input/1 -> iq_ref/1
  Constant/1 -> theta_fd/1

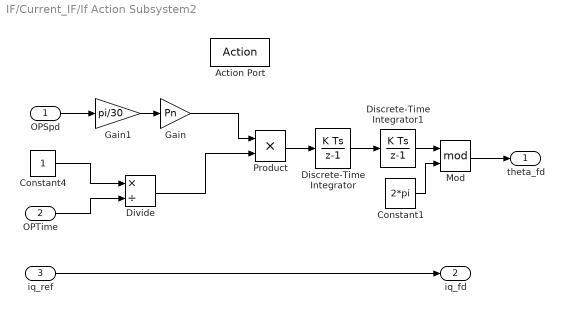
== system IF/Current_IF/If Action Subsystem2 ==
  OPSpd : Inport  OutDataTypeStr=single  PortDimensions=1
  OPTime : Inport  Port=2  OutDataTypeStr=single  PortDimensions=1
  iq_ref : Inport  Port=3
  Action Port : ActionPort  ActionPortLabel=case [ 3 ]:
  Constant1 : Constant  Value=2*pi  OutDataTypeStr=single
  Constant4 : Constant  OutDataTypeStr=single
  Discrete-Time Integrator : DiscreteIntegrator  SampleTime=-1  ICPrevOutput=DiscIntNeverNeededParam  ICPrevScaledInput=DiscIntNeverNeededParam
  Discrete-Time Integrator1 : DiscreteIntegrator  SampleTime=-1  ICPrevOutput=DiscIntNeverNeededParam  ICPrevScaledInput=DiscIntNeverNeededParam
  Divide : Product  Inputs=*/  OutDataTypeStr=single
  Gain : Gain  Gain=Pn
  Gain1 : Gain  Gain=pi/30  OutDataTypeStr=single
  Mod : Math  Operator=mod
  Product : Product  OutDataTypeStr=single
  theta_fd : Outport
  iq_fd : Outport  Port=2
  wires:
  iq_ref/1 -> iq_fd/1
  Constant4/1 -> Divide/1
  Constant1/1 -> Mod/2
  Discrete-Time Integrator1/1 -> Mod/1
  Gain1/1 -> Gain/1
  Divide/1 -> Product/2
  Discrete-Time Integrator/1 -> Discrete-Time Integrator1/1
  Mod/1 -> theta_fd/1
  Gain/1 -> Product/1
  Product/1 -> Discrete-Time Integrator/1
  OPSpd/1 -> Gain1/1
  OPTime/1 -> Divide/2

== system IF/Current_IF/If Action Subsystem3 ==
  OPSpd : Inport  OutDataTypeStr=single  PortDimensions=1
  iq_ref : Inport  Port=2
  Action Port : ActionPort  ActionPortLabel=case [ 4 ]:
  Constant1 : Constant  Value=2*pi  OutDataTypeStr=single
  Discrete-Time Integrator1 : DiscreteIntegrator  SampleTime=-1  ICPrevOutput=DiscIntNeverNeededParam  ICPrevScaledInput=DiscIntNeverNeededParam
  Gain : Gain  Gain=Pn
  Gain1 : Gain  Gain=pi/30  OutDataTypeStr=single
  Mod : Math  Operator=mod
  theta_fd : Outport
  iq_fd : Outport  Port=2
  wires:
  iq_ref/1 -> iq_fd/1
  OPSpd/1 -> Gain1/1
  Discrete-Time Integrator1/1 -> Mod/1
  Constant1/1 -> Mod/2
  Gain/1 -> Discrete-Time Integrator1/1
  Gain1/1 -> Gain/1
  Mod/1 -> theta_fd/1

== system IF/Current_IF/Park ==
  note: id = ialpha*cos(theta)+ibeta*sin(theta);
      | iq = -ialpha*sin(theta)+ibeta*cos(theta);
  ialpha : Inport  OutDataTypeStr=single
  ibeta : Inport  Port=2  OutDataTypeStr=single
  theta_sin : Inport  Port=3  OutDataTypeStr=single
  theta_cos : Inport  Port=4  OutDataTypeStr=single
  Add : Sum  OutDataTypeStr=single  AccumDataTypeStr=single
  Add1 : Sum  Inputs=-+  OutDataTypeStr=single  AccumDataTypeStr=single
  Product{,1..3} (4 alike) : Product  OutDataTypeStr=single
  id : Outport  OutDataTypeStr=single
  iq : Outport  Port=2  OutDataTypeStr=single
  wires:
  theta_cos/1 -> Product/2, Product3/2
  ibeta/1 -> Product1/1, Product3/1
  Product1/1 -> Add/2
  Add1/1 -> iq/1
  Add/1 -> id/1
  Product3/1 -> Add1/2
  ialpha/1 -> Product/1, Product2/1
  Product2/1 -> Add1/1
  Product/1 -> Add/1
  theta_sin/1 -> Product1/2, Product2/2

== system IF/Current_IF/SVPWM ==
  Valpha : Inport  OutDataTypeStr=single
  Vbeta : Inport  Port=2  OutDataTypeStr=single
  v_bus : Inport  Port=3  OutDataTypeStr=single
  AntiClark : Subsystem
  Constant : Constant  Value=0.5  OutDataTypeStr=single
  Divide : Product  Inputs=*/  OutDataTypeStr=single
  Gain : Gain  Gain=-1  OutDataTypeStr=single
  Mux : Mux  Inputs=3
  PWM_HalfPeriod : Gain  Gain=8000  OutDataTypeStr=single
  Sum : Sum  Inputs=++|  OutDataTypeStr=single
  Sum1 : Sum  Inputs=|++  OutDataTypeStr=single
  ei_t : Subsystem
  tABC : Outport  OutDataTypeStr=single
  wires:
  Gain/1 -> Divide/1
  v_bus/1 -> Divide/2
  PWM_HalfPeriod/1 -> tABC/1
  Sum1/1 -> PWM_HalfPeriod/1
  Constant/1 -> Sum1/2
  Divide/1 -> Sum1/1
  Mux/1 -> ei_t/1(Vabc), Sum/2
  Sum/1 -> Gain/1
  AntiClark/3(Vc) -> Mux/3
  AntiClark/2(Vb) -> Mux/2
  AntiClark/1(Va) -> Mux/1
  ei_t/1(ei_t) -> Sum/1
  Vbeta/1 -> AntiClark/2(Vbeta)
  Valpha/1 -> AntiClark/1(Valpha)

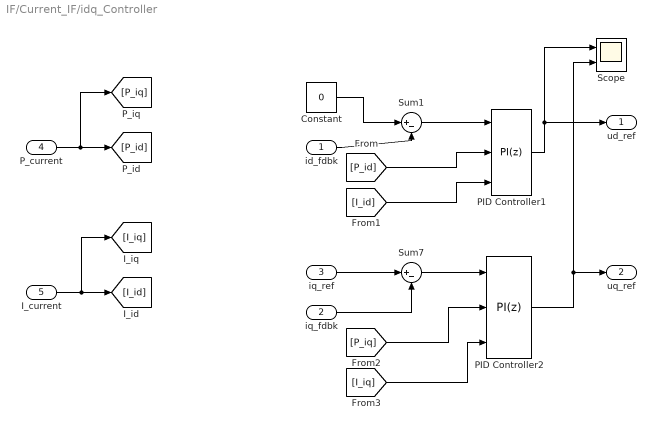
== system IF/Current_IF/idq_Controller ==
  id_fdbk : Inport  OutDataTypeStr=single
  iq_fdbk : Inport  Port=2  OutDataTypeStr=single
  iq_ref : Inport  Port=3  OutDataTypeStr=single
  P_current : Inport  Port=4
  I_current : Inport  Port=5
  Constant : Constant  Value=0  OutDataTypeStr=single
  PID Controller1 : slpidlib/PID Controller  Controller=PI  Form=Parallel  TimeDomain=Discrete-time  UseExternalTs=off  SampleTime=-1  IntegratorMethod=Forward Euler  FilterMethod=Forward Euler  ControllerParametersSource=external  P=curr_d_kp  I=curr_d_ki  UseKiTs=off  D=0  UseExternalDerivativeSource=off  N=100  UseFilter=on  TunerSelectOption=Transfer Function Based (PID Tuner App)  InitialConditionSource=internal  InitialConditionForIntegrator=0  InitialConditionForFilter=0  DifferentiatorICPrevScaledInput=0  ExternalReset=none  TrackingMode=off  Kt=1  LimitOutput=on  SatLimitsSource=internal  UpperSaturationLimit=Udc*0.9/sqrt(3)  LowerSaturationLimit=-Udc*0.9/sqrt(3)  LinearizeAsGain=on  AntiWindupMode=clamping  Kb=1  LimitIntegrator=off  UpperIntegratorSaturationLimit=inf  LowerIntegratorSaturationLimit=-inf  PGainOutDataTypeStr=single  PProdOutDataTypeStr=single  POutMin=[]  POutMax=[]  IGainOutDataTypeStr=single  IProdOutDataTypeStr=single  IOutMin=[]  IOutMax=[]  DOutMin=[]  DOutMax=[]  NOutMin=[]  NOutMax=[]  SumOutDataTypeStr=single  SumOutMin=[]  SumOutMax=[]  SaturationOutDataTypeStr=single  SaturationOutMin=[]  SaturationOutMax=[]  PParamMin=[]  PParamMax=[]  IParamMin=[]  IParamMax=[]  DParamMin=[]  DParamMax=[]  NParamMin=[]  NParamMax=[]  KbParamMin=[]  KbParamMax=[]  KtParamMin=[]  KtParamMax=[]  KbOutMin=[]  KbOutMax=[]  KtOutMin=[]  KtOutMax=[]  IntegratorOutMin=[]  IntegratorOutMax=[]  FilterOutMin=[]  FilterOutMax=[]  SumI1OutMin=[]  SumI1OutMax=[]  SumI2OutMin=[]  SumI2OutMax=[]  SumI3OutMin=[]  SumI3OutMax=[]  SumI4OutMin=[]  SumI4OutMax=[]  SumDOutMin=[]  SumDOutMax=[]  DifferentiatorOutMin=[]  DifferentiatorOutMax=[]  FilterDiffOutCoefMin=[]  FilterDiffOutCoefMax=[]  ReciprocalOutMin=[]  ReciprocalOutMax=[]  SumDenOutMin=[]  SumDenOutMax=[]  SumNumOutMin=[]  SumNumOutMax=[]  DivideOutMin=[]  DivideOutMax=[]  UdiffTsProdOutMin=[]  UdiffTsProdOutMax=[]  NTsProdOutMin=[]  NTsProdOutMax=[]  UintegralTsProdOutMin=[]  UintegralTsProdOutMax=[]  UngainTsProdOutMin=[]  UngainTsProdOutMax=[]  ClampingZeroOutDataTypeStr=Inherit: Inherit via back propagation  ClampingZeroOutMin=[]  ClampingZeroOutMax=[]  FilterDenConstantOutDataTypeStr=Inherit: Inherit via back propagation  FilterDenConstantOutMin=[]  FilterDenConstantOutMax=[]  PCopyOutDataTypeStr=Inherit: Inherit via back propagation  PCopyOutMin=[]  PCopyOutMax=[]  NCopyOutDataTypeStr=Inherit: Inherit via back propagation  NCopyOutMin=[]  NCopyOutMax=[]  IntegratorContinuousStateAttributes=''  IntegratorStateMustResolveToSignalObject=off  IntegratorRTWStateStorageClass=Auto  FilterContinuousStateAttributes=''  FilterStateMustResolveToSignalObject=off  FilterRTWStateStorageClass=Auto  ParallelPVariant=ExternalParameters  IdealPVariant=Disabled  IVariant=ExternalParameters  DVariant=Disabled  IntegratorVariant=Discrete  SatVariant=Enabled  AWVariant=DiscClampingParallel  PCopyVariant=Disabled  TRVariant=Disabled  FdbkBlocksVariant=Forward  IdealPFdbkVariant=Disabled  SatFdbkVariant=Disabled  DerivativeFilterVariant=Disabled  NVariant=Disabled  NCopyVariant=Disabled_SignalSpec  FilterICVariant=Disabled  IntegratorICVariant=InternalICs  ExternalResetVariant=Disabled  TRSumVariant=Passthrough  SumFdbkVariant=Disabled  SumVariant=Sum_PI  TsampFilterVariant=InternalTs  TsampNgainVariant=Passthrough  TsampIntegralVariant=Disabled_SignalSpec  ExternalSaturationOutDataTypeStr=Inherit: Same as second input  DerivativeSourceVariant=Disabled
  PID Controller2 : slpidlib/PID Controller  Controller=PI  Form=Parallel  TimeDomain=Discrete-time  UseExternalTs=off  SampleTime=-1  IntegratorMethod=Forward Euler  FilterMethod=Forward Euler  ControllerParametersSource=external  P=curr_q_kp  I=curr_q_ki  UseKiTs=off  D=0  UseExternalDerivativeSource=off  N=100  UseFilter=on  TunerSelectOption=Transfer Function Based (PID Tuner App)  InitialConditionSource=internal  InitialConditionForIntegrator=0  InitialConditionForFilter=0  DifferentiatorICPrevScaledInput=0  ExternalReset=none  TrackingMode=off  Kt=1  LimitOutput=on  SatLimitsSource=internal  UpperSaturationLimit=Udc*0.9/sqrt(3)  LowerSaturationLimit=-Udc*0.9/sqrt(3)  LinearizeAsGain=on  AntiWindupMode=clamping  Kb=1  LimitIntegrator=off  UpperIntegratorSaturationLimit=inf  LowerIntegratorSaturationLimit=-inf  PGainOutDataTypeStr=single  PProdOutDataTypeStr=single  POutMin=[]  POutMax=[]  IGainOutDataTypeStr=single  IProdOutDataTypeStr=single  IOutMin=[]  IOutMax=[]  DOutMin=[]  DOutMax=[]  NOutMin=[]  NOutMax=[]  SumOutDataTypeStr=single  SumOutMin=[]  SumOutMax=[]  SaturationOutDataTypeStr=single  SaturationOutMin=[]  SaturationOutMax=[]  PParamMin=[]  PParamMax=[]  IParamMin=[]  IParamMax=[]  DParamMin=[]  DParamMax=[]  NParamMin=[]  NParamMax=[]  KbParamMin=[]  KbParamMax=[]  KtParamMin=[]  KtParamMax=[]  KbOutMin=[]  KbOutMax=[]  KtOutMin=[]  KtOutMax=[]  IntegratorOutMin=[]  IntegratorOutMax=[]  FilterOutMin=[]  FilterOutMax=[]  SumI1OutMin=[]  SumI1OutMax=[]  SumI2OutMin=[]  SumI2OutMax=[]  SumI3OutMin=[]  SumI3OutMax=[]  SumI4OutMin=[]  SumI4OutMax=[]  SumDOutMin=[]  SumDOutMax=[]  DifferentiatorOutMin=[]  DifferentiatorOutMax=[]  FilterDiffOutCoefMin=[]  FilterDiffOutCoefMax=[]  ReciprocalOutMin=[]  ReciprocalOutMax=[]  SumDenOutMin=[]  SumDenOutMax=[]  SumNumOutMin=[]  SumNumOutMax=[]  DivideOutMin=[]  DivideOutMax=[]  UdiffTsProdOutMin=[]  UdiffTsProdOutMax=[]  NTsProdOutMin=[]  NTsProdOutMax=[]  UintegralTsProdOutMin=[]  UintegralTsProdOutMax=[]  UngainTsProdOutMin=[]  UngainTsProdOutMax=[]  ClampingZeroOutDataTypeStr=Inherit: Inherit via back propagation  ClampingZeroOutMin=[]  ClampingZeroOutMax=[]  FilterDenConstantOutDataTypeStr=Inherit: Inherit via back propagation  FilterDenConstantOutMin=[]  FilterDenConstantOutMax=[]  PCopyOutDataTypeStr=Inherit: Inherit via back propagation  PCopyOutMin=[]  PCopyOutMax=[]  NCopyOutDataTypeStr=Inherit: Inherit via back propagation  NCopyOutMin=[]  NCopyOutMax=[]  IntegratorContinuousStateAttributes=''  IntegratorStateMustResolveToSignalObject=off  IntegratorRTWStateStorageClass=Auto  FilterContinuousStateAttributes=''  FilterStateMustResolveToSignalObject=off  FilterRTWStateStorageClass=Auto  ParallelPVariant=ExternalParameters  IdealPVariant=Disabled  IVariant=ExternalParameters  DVariant=Disabled  IntegratorVariant=Discrete  SatVariant=Enabled  AWVariant=DiscClampingParallel  PCopyVariant=Disabled  TRVariant=Disabled  FdbkBlocksVariant=Forward  IdealPFdbkVariant=Disabled  SatFdbkVariant=Disabled  DerivativeFilterVariant=Disabled  NVariant=Disabled  NCopyVariant=Disabled_SignalSpec  FilterICVariant=Disabled  IntegratorICVariant=InternalICs  ExternalResetVariant=Disabled  TRSumVariant=Passthrough  SumFdbkVariant=Disabled  SumVariant=Sum_PI  TsampFilterVariant=InternalTs  TsampNgainVariant=Passthrough  TsampIntegralVariant=Disabled_SignalSpec  ExternalSaturationOutDataTypeStr=Inherit: Same as second input  DerivativeSourceVariant=Disabled
  Scope : Scope  NumInputPorts=2
  Sum1 : Sum  Inputs=|+-  OutDataTypeStr=single  AccumDataTypeStr=single
  Sum7 : Sum  Inputs=|+-  OutDataTypeStr=single  AccumDataTypeStr=single
  ud_ref : Outport  OutDataTypeStr=single
  uq_ref : Outport  Port=2  OutDataTypeStr=single
  wires:
  id_fdbk/1 -> Sum1/2
  Constant/1 -> Sum1/1
  iq_fdbk/1 -> Sum7/2
  Sum1/1 -> PID Controller1/1
  Sum7/1 -> PID Controller2/1
  PID Controller1/1 -> Scope/1, ud_ref/1
  PID Controller2/1 -> Scope/2, uq_ref/1
  iq_ref/1 -> Sum7/1
  [P_id] -> PID Controller1/2
  [I_id] -> PID Controller1/3
  [P_iq] -> PID Controller2/2
  [I_iq] -> PID Controller2/3
  P_current/1 -> [P_id], [P_iq]
  I_current/1 -> [I_iq], [I_id]

== system IF/Current_IF1/Clark ==
  note: ialpha = ia*2/3-(ib+ic)/3;
      | ibeta = (ib-ic)*sqrt(3)/3;
  ia : Inport  OutDataTypeStr=single
  ib : Inport  Port=2  OutDataTypeStr=single
  ic : Inport  Port=3  OutDataTypeStr=single
  Add : Sum  OutDataTypeStr=single  AccumDataTypeStr=single
  Add1 : Sum  Inputs=+-  OutDataTypeStr=single  AccumDataTypeStr=single
  Add2 : Sum  Inputs=+-  OutDataTypeStr=single  AccumDataTypeStr=single
  Gain : Gain  Gain=2/3  ParamDataTypeStr=single
  Gain1 : Gain  Gain=1/3  ParamDataTypeStr=single
  Gain2 : Gain  Gain=sqrt(3)/3  ParamDataTypeStr=single
  ialpha : Outport  OutDataTypeStr=single
  ibeta : Outport  Port=2  OutDataTypeStr=single
  wires:
  Add1/1 -> ialpha/1
  ia/1 -> Gain/1
  Gain2/1 -> ibeta/1
  ib/1 -> Add/1, Add2/1
  Gain/1 -> Add1/1
  Add2/1 -> Gain2/1
  Add/1 -> Gain1/1
  ic/1 -> Add/2, Add2/2
  Gain1/1 -> Add1/2

== system IF/Current_IF1/If Action Subsystem ==
  Action Port : ActionPort  ActionPortLabel=case [ 1 ]:
  Constant : Constant  Value=0  OutDataTypeStr=single
  Constant1 : Constant  Value=0  OutDataTypeStr=single
  theta_fd : Outport
  iq_ref : Outport  Port=2
  wires:
  Constant1/1 -> iq_ref/1
  Constant/1 -> theta_fd/1

== system IF/Current_IF1/If Action Subsystem1 ==
  Input : Inport
  Action Port : ActionPort  ActionPortLabel=case [ 2 ]:
  Constant : Constant  Value=0  OutDataTypeStr=single
  theta_fd : Outport
  iq_ref : Outport  Port=2
  wires:
  Input/1 -> iq_ref/1
  Constant/1 -> theta_fd/1

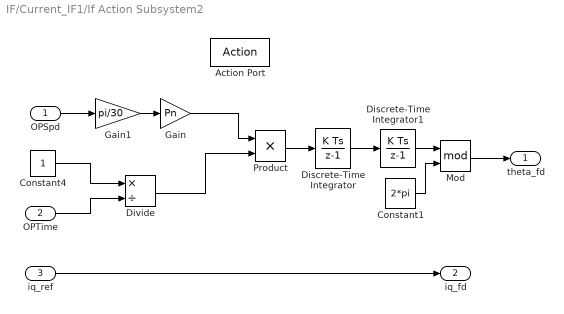
== system IF/Current_IF1/If Action Subsystem2 ==
  OPSpd : Inport  OutDataTypeStr=single  PortDimensions=1
  OPTime : Inport  Port=2  OutDataTypeStr=single  PortDimensions=1
  iq_ref : Inport  Port=3
  Action Port : ActionPort  ActionPortLabel=case [ 3 ]:
  Constant1 : Constant  Value=2*pi  OutDataTypeStr=single
  Constant4 : Constant  OutDataTypeStr=single
  Discrete-Time Integrator : DiscreteIntegrator  SampleTime=-1  ICPrevOutput=DiscIntNeverNeededParam  ICPrevScaledInput=DiscIntNeverNeededParam
  Discrete-Time Integrator1 : DiscreteIntegrator  SampleTime=-1  ICPrevOutput=DiscIntNeverNeededParam  ICPrevScaledInput=DiscIntNeverNeededParam
  Divide : Product  Inputs=*/  OutDataTypeStr=single
  Gain : Gain  Gain=Pn
  Gain1 : Gain  Gain=pi/30  OutDataTypeStr=single
  Mod : Math  Operator=mod
  Product : Product  OutDataTypeStr=single
  theta_fd : Outport
  iq_fd : Outport  Port=2
  wires:
  iq_ref/1 -> iq_fd/1
  Constant4/1 -> Divide/1
  Constant1/1 -> Mod/2
  Discrete-Time Integrator1/1 -> Mod/1
  Gain1/1 -> Gain/1
  Divide/1 -> Product/2
  Discrete-Time Integrator/1 -> Discrete-Time Integrator1/1
  Mod/1 -> theta_fd/1
  Gain/1 -> Product/1
  Product/1 -> Discrete-Time Integrator/1
  OPSpd/1 -> Gain1/1
  OPTime/1 -> Divide/2

== system IF/Current_IF1/If Action Subsystem3 ==
  OPSpd : Inport  OutDataTypeStr=single  PortDimensions=1
  iq_ref : Inport  Port=2
  Action Port : ActionPort  ActionPortLabel=case [ 4 ]:
  Constant1 : Constant  Value=2*pi  OutDataTypeStr=single
  Discrete-Time Integrator1 : DiscreteIntegrator  SampleTime=-1  ICPrevOutput=DiscIntNeverNeededParam  ICPrevScaledInput=DiscIntNeverNeededParam
  Gain : Gain  Gain=Pn
  Gain1 : Gain  Gain=pi/30  OutDataTypeStr=single
  Mod : Math  Operator=mod
  theta_fd : Outport
  iq_fd : Outport  Port=2
  wires:
  iq_ref/1 -> iq_fd/1
  OPSpd/1 -> Gain1/1
  Discrete-Time Integrator1/1 -> Mod/1
  Constant1/1 -> Mod/2
  Gain/1 -> Discrete-Time Integrator1/1
  Gain1/1 -> Gain/1
  Mod/1 -> theta_fd/1

== system IF/Current_IF1/Park ==
  note: id = ialpha*cos(theta)+ibeta*sin(theta);
      | iq = -ialpha*sin(theta)+ibeta*cos(theta);
  ialpha : Inport  OutDataTypeStr=single
  ibeta : Inport  Port=2  OutDataTypeStr=single
  theta_sin : Inport  Port=3  OutDataTypeStr=single
  theta_cos : Inport  Port=4  OutDataTypeStr=single
  Add : Sum  OutDataTypeStr=single  AccumDataTypeStr=single
  Add1 : Sum  Inputs=-+  OutDataTypeStr=single  AccumDataTypeStr=single
  Product{,1..3} (4 alike) : Product  OutDataTypeStr=single
  id : Outport  OutDataTypeStr=single
  iq : Outport  Port=2  OutDataTypeStr=single
  wires:
  theta_cos/1 -> Product/2, Product3/2
  ibeta/1 -> Product1/1, Product3/1
  Product1/1 -> Add/2
  Add1/1 -> iq/1
  Add/1 -> id/1
  Product3/1 -> Add1/2
  ialpha/1 -> Product/1, Product2/1
  Product2/1 -> Add1/1
  Product/1 -> Add/1
  theta_sin/1 -> Product1/2, Product2/2
